simulink model "ej2b_Qi"  (R2021a)
settings: Solver=VariableStepAuto  StartTime=0.0  StopTime=2000  RelTol=1e-3
values from neighbouring files (symbols this model uses):
  h0 = h0_valores(i)    [EJ1.m]    (also in EJ2.m = 0.45; ej1b.m = 0.45; ej1e.m; ej2a.m = 0.45)
  Q_i = 0.0001333    [EJ1.m]    (also in EJ2.m; ej1b.m; ej1e.m; ej2a.m)
  u0 = Q_i / (A_o * sqrt(2 * g * h0))    [EJ1.m]    (also in EJ2.m; ej1b.m; ej1e.m; ej2a.m)
libraries: cstblocks x3
settings Model: Creator=franc  LastModifiedBy=facun

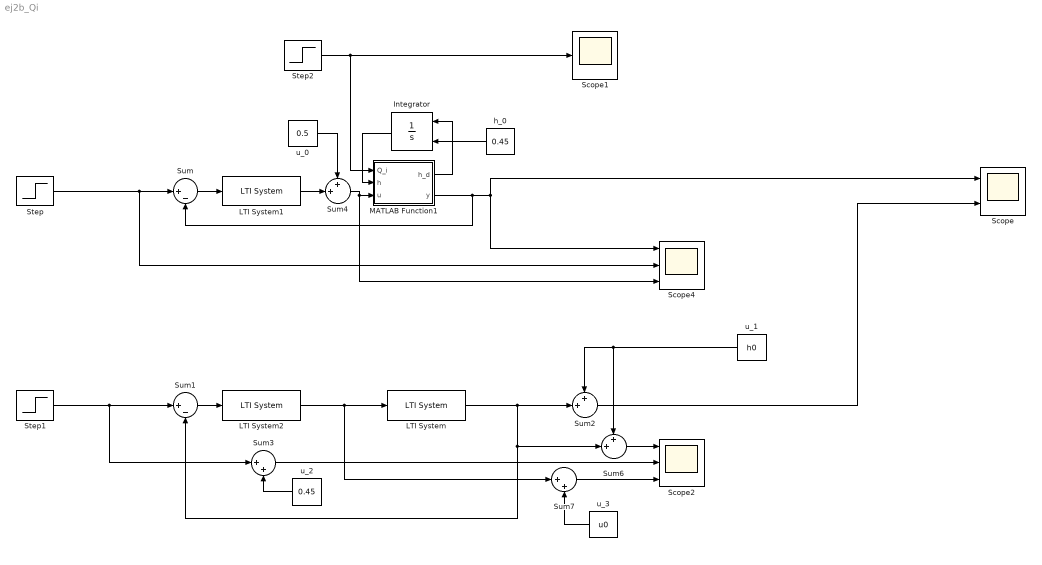
== system ej2b_Qi ==
  Integrator : Integrator  InitialConditionSource=external
  LTI System : cstblocks/LTI System  sys=Pmp  IC=[]
  LTI System1 : cstblocks/LTI System  sys=Cs  IC=[]
  LTI System2 : cstblocks/LTI System  sys=Cs  IC=[]
  MATLAB Function1 : MATLAB Function  TreatAsAtomicUnit=on
  Scope : Scope  NumInputPorts=2
  Scope1 : Scope
  Scope2 : Scope  NumInputPorts=3
  Scope4 : Scope  NumInputPorts=3
  Step : Step  Time=300  Before=0.45  After=0.35  SampleTime=0
  Step1 : Step  Time=1000  After=0.1  SampleTime=0
  Step2 : Step  Time=600  Before=Q_i  After=Q_i*0.9  SampleTime=0
  Sum : Sum  Inputs=|+-
  Sum1 : Sum  Inputs=|+-
  Sum2 : Sum  Inputs=++|
  Sum3 : Sum  Inputs=|++
  Sum4 : Sum  Inputs=++|
  Sum6 : Sum  Inputs=++|
  Sum7 : Sum  Inputs=|++
  h_0 : Constant  Value=0.45
  u_0 : Constant  Value=0.5
  u_1 : Constant  Value=h0
  u_2 : Constant  Value=0.45
  u_3 : Constant  Value=u0
  wires:
  Step/1 -> Scope4/2, Sum/1
  MATLAB Function1/2(y) -> Scope/1, Scope4/1, Sum/2
  MATLAB Function1/1(h_d) -> Integrator/1
  h_0/1 -> Integrator/2
  Sum1/1 -> LTI System2/1
  Step1/1 -> Sum3/1, Sum1/1
  Sum/1 -> LTI System1/1
  u_0/1 -> Sum4/1
  LTI System1/1 -> Sum4/2
  Sum4/1 -> Scope4/3, MATLAB Function1/3(u)
  Sum2/1 -> Scope/2
  u_1/1 -> Sum6/1, Sum2/1
  LTI System2/1 -> Sum7/1, LTI System/1
  Sum6/1 -> Scope2/1
  LTI System/1 -> Sum2/2, Sum1/2, Sum6/2
  u_3/1 -> Sum7/2
  Sum7/1 -> Scope2/3
  u_2/1 -> Sum3/2
  Sum3/1 -> Scope2/2
  Integrator/1 -> MATLAB Function1/2(h)
  Step2/1 -> MATLAB Function1/1(Q_i), Scope1/1

== matlab function ej2b_Qi/MATLAB Function1 ==
  data: Q_i input; h input; h_d output; u input; y output
function [h_d, y] = fcn(Q_i, h, u)
    g = 9.8;        %En metros sobre segundo cuadrado
    H = 0.9;        %En metros
    L_s = 0.4;      %En metros
    L_i = 0.1;      %En metros
    d2 = 10.65e-3;
    A_o = pi * (d2 / 2)^2;

    h_d = (H^2 * (Q_i - A_o * sqrt(2*g*h)*u))/(h^2*(L_s-L_i)^2 + 2*h*L_i*(L_s-L_i)*H+L_i^2*H^2);
    y = h;
end
